simulink model "scheme1"  (R2014a)
settings: Solver=ode45  StartTime=0.0  StopTime=0.4  MaxStep=0.001  MinStep=0.0001  RelTol=1e-3
settings Model: Creator=User  LastModifiedBy=trigg

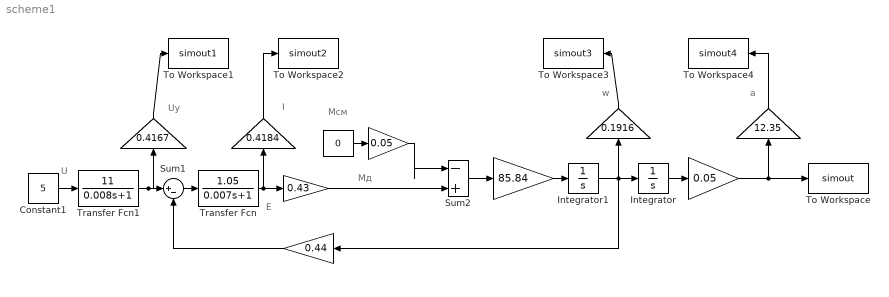
== system scheme1 ==
  note: E
  note: a
  note: w
  note: Мд
  note: Mсм
  note: I
  note: Uy
  note: U
  " " : Constant  Value=0
  "  " : Gain  Gain=0.4167
  "   " : Gain  Gain=0.43
  "    " : Gain  Gain=0.44
  "     " : Gain  Gain=0.05
  "      " : Gain  Gain=0.4184
  "       " : Gain  Gain=85.84
  "        " : Gain  Gain=0.05
  "         " : Gain  Gain=0.1916
  "               " : Gain  Gain=12.35
  Constant1 : Constant  Value=5
  Integrator : Integrator
  Integrator1 : Integrator
  Sum1 : Sum  Inputs=|+-
  Sum2 : Sum  Inputs=|-+
  To Workspace : ToWorkspace  VariableName=simout  SaveFormat=Timeseries  SampleTime=-1
  To Workspace1 : ToWorkspace  VariableName=simout1  SaveFormat=Timeseries  SampleTime=-1
  To Workspace2 : ToWorkspace  VariableName=simout2  SaveFormat=Timeseries  SampleTime=-1
  To Workspace3 : ToWorkspace  VariableName=simout3  SaveFormat=Timeseries  SampleTime=-1
  To Workspace4 : ToWorkspace  VariableName=simout4  SaveFormat=Timeseries  SampleTime=-1
  Transfer Fcn : TransferFcn  Numerator=[1.05]  Denominator=[0.007 1]
  Transfer Fcn1 : TransferFcn  Numerator=[11]  Denominator=[0.008 1]
  wires:
  Constant1/1 -> Transfer Fcn1/1
  Transfer Fcn1/1 -> Sum1/1, "  "/1
  Transfer Fcn/1 -> "   "/1, "      "/1
  "   "/1 -> Sum2/2
  " "/1 -> "     "/1
  "     "/1 -> Sum2/1
  "       "/1 -> Integrator1/1
  Integrator1/1 -> "    "/1, Integrator/1, "         "/1
  "    "/1 -> Sum1/2
  Sum1/1 -> Transfer Fcn/1
  Integrator/1 -> "        "/1
  "        "/1 -> To Workspace/1, "               "/1
  Sum2/1 -> "       "/1
  "  "/1 -> To Workspace1/1
  "      "/1 -> To Workspace2/1
  "         "/1 -> To Workspace3/1
  "               "/1 -> To Workspace4/1
